simulink model "DR_Screening_Simulink"  (R2026a)
settings: Solver=FixedStepDiscrete  StopTime=100  FixedStep=1
settings Model: Creator=LENOVO  LastModifiedBy=LENOVO

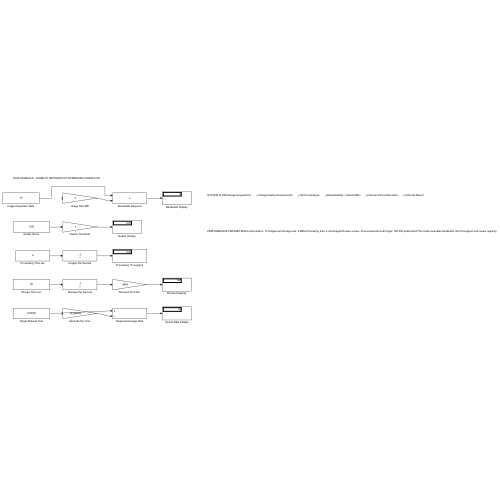
[thumbnail: Simulink's stored preview of the top-level diagram]
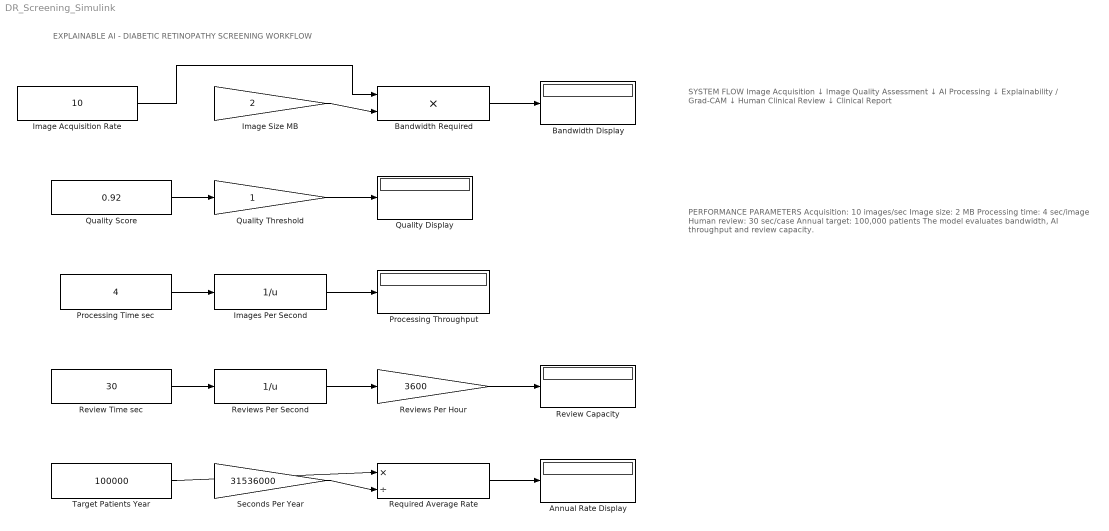
== system DR_Screening_Simulink ==
  note: EXPLAINABLE AI - DIABETIC RETINOPATHY SCREENING WORKFLOW
  note: SYSTEM FLOW\nImage Acquisition\n ↓\nImage Quality Assessment\n ↓\nAI Processing\n ↓\nExplainability / Grad-CAM\n ↓\nHuman Clinical Review\n ↓\nClinical Report
  note: PERFORMANCE PARAMETERS\n\nAcquisition: 10 images/sec\nImage size: 2 MB\nProcessing time: 4 sec/image\nHuman review: 30 sec/case\nAnnual target: 100,000 patients\n\nThe model evaluates bandwidth,\nAI throughput and review capacity.
  Annual Rate Display : Display
  Bandwidth Display : Display
  Bandwidth Required : Product
  Image Acquisition Rate : Constant  Value=10
  Image Size MB : Gain  Gain=2
  Images Per Second : Math  Operator=reciprocal
  Processing Throughput : Display
  Processing Time sec : Constant  Value=4
  Quality Display : Display
  Quality Score : Constant  Value=0.92
  Quality Threshold : Gain
  Required Average Rate : Product  Inputs=*/
  Review Capacity : Display
  Review Time sec : Constant  Value=30
  Reviews Per Hour : Gain  Gain=3600
  Reviews Per Second : Math  Operator=reciprocal
  Seconds Per Year : Gain  Gain=31536000
  Target Patients Year : Constant  Value=100000
  wires:
  Image Acquisition Rate/1 -> Bandwidth Required/1
  Image Size MB/1 -> Bandwidth Required/2
  Bandwidth Required/1 -> Bandwidth Display/1
  Quality Score/1 -> Quality Threshold/1
  Quality Threshold/1 -> Quality Display/1
  Processing Time sec/1 -> Images Per Second/1
  Images Per Second/1 -> Processing Throughput/1
  Review Time sec/1 -> Reviews Per Second/1
  Reviews Per Second/1 -> Reviews Per Hour/1
  Reviews Per Hour/1 -> Review Capacity/1
  Target Patients Year/1 -> Required Average Rate/1
  Seconds Per Year/1 -> Required Average Rate/2
  Required Average Rate/1 -> Annual Rate Display/1
